simulink model "SoftwareArchitecture"  (R2024a)
settings: Solver=FixedStepDiscrete  StartTime=0.0  StopTime=10.0  RelTol=1e-3
settings Model: Creator=njsne  LastModifiedBy=njsne

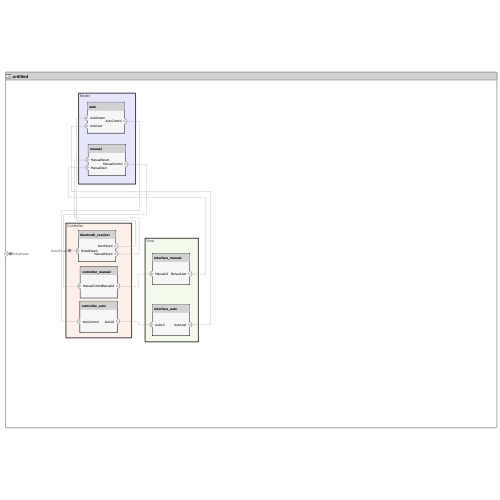
[thumbnail: Simulink's stored preview of the top-level diagram]
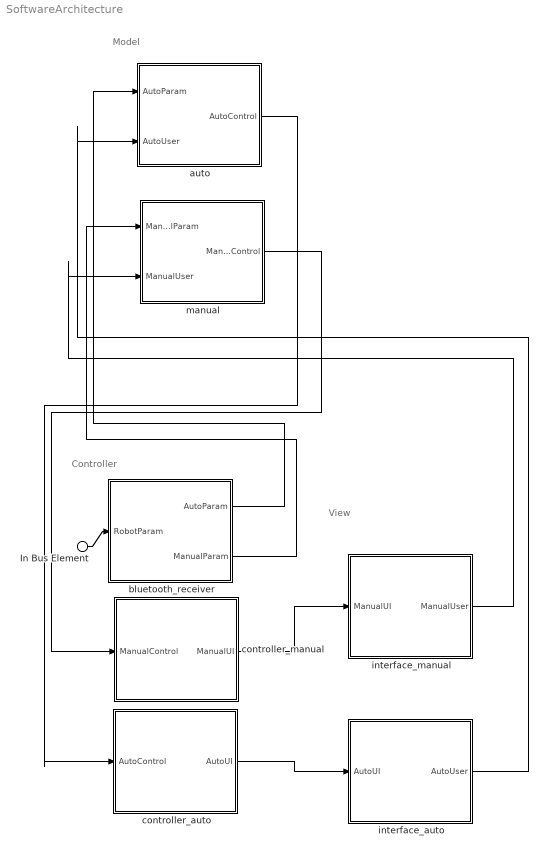
== system SoftwareArchitecture ==
  note: Model
  note: Controller
  note: View
  In Bus Element : Inport  PortName=RobotParam
  auto : Subsystem
      settings: PortSchema="{\"entries\":[{\"content\":{\"headerSize\":26,\"margin\":15,\"minimumSpacing\":25,\"sides\":[{\"content\":{\"connectorIds\":[\"In1\",\"In2\"]},\"type\":\"ConnectorPlacement.EquallySpacedRectSide\",\"uuid\":\"f355d6d0-cf58-497d-af4c-3e4dcc6a73b6\"},{\"content\":{\"connectorIds\":[\"Out1\"],\"side\":\"RIGHT\"},\"type\":\"ConnectorPlacement.EquallySpacedRectSide\",\"uuid\":\"26958e8c-f185-4cf9-b08a-6b963fcd1ab7\"},{\"content\":{\"side\":\"TOP\"},\"type\":\"ConnectorPlacement.EquallySpacedRectSide\",\"uuid\":\"bb7e5bb3-6807-4390-828c-0753e6f4db2d\"}]},\"type\":\"ConnectorPlacement.EquallySpacedConnector\",\"uuid\":\"9cb3c599-3bd4-42ed-97e1-2535c9f88a3a\"}],\"packageUris\":[\"http://schema.mathworks.com/mf0/Connector/R2020b\"],\"version\":\"1.0\"}"
  bluetooth_receiver : Subsystem
      settings: PortSchema="{\"entries\":[{\"content\":{\"headerSize\":26,\"margin\":15,\"minimumSpacing\":25,\"sides\":[{\"content\":{\"connectorIds\":[\"In1\"]},\"type\":\"ConnectorPlacement.EquallySpacedRectSide\",\"uuid\":\"f355d6d0-cf58-497d-af4c-3e4dcc6a73b6\"},{\"content\":{\"connectorIds\":[\"Out1\",\"Out2\"],\"side\":\"RIGHT\"},\"type\":\"ConnectorPlacement.EquallySpacedRectSide\",\"uuid\":\"26958e8c-f185-4cf9-b08a-6b963fcd1ab7\"},{\"content\":{\"side\":\"TOP\"},\"type\":\"ConnectorPlacement.EquallySpacedRectSide\",\"uuid\":\"bb7e5bb3-6807-4390-828c-0753e6f4db2d\"}]},\"type\":\"ConnectorPlacement.EquallySpacedConnector\",\"uuid\":\"9cb3c599-3bd4-42ed-97e1-2535c9f88a3a\"}],\"packageUris\":[\"http://schema.mathworks.com/mf0/Connector/R2020b\"],\"version\":\"1.0\"}"
  controller_auto : Subsystem
      settings: PortSchema="{\"entries\":[{\"content\":{\"headerSize\":26,\"margin\":15,\"minimumSpacing\":25,\"sides\":[{\"content\":{\"connectorIds\":[\"In1\"]},\"type\":\"ConnectorPlacement.EquallySpacedRectSide\",\"uuid\":\"f355d6d0-cf58-497d-af4c-3e4dcc6a73b6\"},{\"content\":{\"connectorIds\":[\"Out1\"],\"side\":\"RIGHT\"},\"type\":\"ConnectorPlacement.EquallySpacedRectSide\",\"uuid\":\"26958e8c-f185-4cf9-b08a-6b963fcd1ab7\"},{\"content\":{\"side\":\"TOP\"},\"type\":\"ConnectorPlacement.EquallySpacedRectSide\",\"uuid\":\"bb7e5bb3-6807-4390-828c-0753e6f4db2d\"}]},\"type\":\"ConnectorPlacement.EquallySpacedConnector\",\"uuid\":\"9cb3c599-3bd4-42ed-97e1-2535c9f88a3a\"}],\"packageUris\":[\"http://schema.mathworks.com/mf0/Connector/R2020b\"],\"version\":\"1.0\"}"
  controller_manual : Subsystem
      settings: PortSchema="{\"entries\":[{\"content\":{\"headerSize\":26,\"margin\":15,\"minimumSpacing\":25,\"sides\":[{\"content\":{\"connectorIds\":[\"In1\"]},\"type\":\"ConnectorPlacement.EquallySpacedRectSide\",\"uuid\":\"f355d6d0-cf58-497d-af4c-3e4dcc6a73b6\"},{\"content\":{\"connectorIds\":[\"Out1\"],\"side\":\"RIGHT\"},\"type\":\"ConnectorPlacement.EquallySpacedRectSide\",\"uuid\":\"26958e8c-f185-4cf9-b08a-6b963fcd1ab7\"},{\"content\":{\"side\":\"TOP\"},\"type\":\"ConnectorPlacement.EquallySpacedRectSide\",\"uuid\":\"bb7e5bb3-6807-4390-828c-0753e6f4db2d\"}]},\"type\":\"ConnectorPlacement.EquallySpacedConnector\",\"uuid\":\"9cb3c599-3bd4-42ed-97e1-2535c9f88a3a\"}],\"packageUris\":[\"http://schema.mathworks.com/mf0/Connector/R2020b\"],\"version\":\"1.0\"}"
  interface_auto : Subsystem
      settings: PortSchema="{\"entries\":[{\"content\":{\"headerSize\":26,\"margin\":15,\"minimumSpacing\":25,\"sides\":[{\"content\":{\"connectorIds\":[\"In1\"]},\"type\":\"ConnectorPlacement.EquallySpacedRectSide\",\"uuid\":\"f355d6d0-cf58-497d-af4c-3e4dcc6a73b6\"},{\"content\":{\"connectorIds\":[\"Out1\"],\"side\":\"RIGHT\"},\"type\":\"ConnectorPlacement.EquallySpacedRectSide\",\"uuid\":\"26958e8c-f185-4cf9-b08a-6b963fcd1ab7\"},{\"content\":{\"side\":\"TOP\"},\"type\":\"ConnectorPlacement.EquallySpacedRectSide\",\"uuid\":\"bb7e5bb3-6807-4390-828c-0753e6f4db2d\"}]},\"type\":\"ConnectorPlacement.EquallySpacedConnector\",\"uuid\":\"9cb3c599-3bd4-42ed-97e1-2535c9f88a3a\"}],\"packageUris\":[\"http://schema.mathworks.com/mf0/Connector/R2020b\"],\"version\":\"1.0\"}"
  interface_manual : Subsystem
      settings: PortSchema="{\"entries\":[{\"content\":{\"headerSize\":26,\"margin\":15,\"minimumSpacing\":25,\"sides\":[{\"content\":{\"connectorIds\":[\"In1\"]},\"type\":\"ConnectorPlacement.EquallySpacedRectSide\",\"uuid\":\"f355d6d0-cf58-497d-af4c-3e4dcc6a73b6\"},{\"content\":{\"connectorIds\":[\"Out1\"],\"side\":\"RIGHT\"},\"type\":\"ConnectorPlacement.EquallySpacedRectSide\",\"uuid\":\"26958e8c-f185-4cf9-b08a-6b963fcd1ab7\"},{\"content\":{\"side\":\"TOP\"},\"type\":\"ConnectorPlacement.EquallySpacedRectSide\",\"uuid\":\"bb7e5bb3-6807-4390-828c-0753e6f4db2d\"}]},\"type\":\"ConnectorPlacement.EquallySpacedConnector\",\"uuid\":\"9cb3c599-3bd4-42ed-97e1-2535c9f88a3a\"}],\"packageUris\":[\"http://schema.mathworks.com/mf0/Connector/R2020b\"],\"version\":\"1.0\"}"
  manual : Subsystem
      settings: PortSchema="{\"entries\":[{\"content\":{\"headerSize\":26,\"margin\":15,\"minimumSpacing\":25,\"sides\":[{\"content\":{\"connectorIds\":[\"In1\",\"In2\"]},\"type\":\"ConnectorPlacement.EquallySpacedRectSide\",\"uuid\":\"f355d6d0-cf58-497d-af4c-3e4dcc6a73b6\"},{\"content\":{\"connectorIds\":[\"Out1\"],\"side\":\"RIGHT\"},\"type\":\"ConnectorPlacement.EquallySpacedRectSide\",\"uuid\":\"26958e8c-f185-4cf9-b08a-6b963fcd1ab7\"},{\"content\":{\"side\":\"TOP\"},\"type\":\"ConnectorPlacement.EquallySpacedRectSide\",\"uuid\":\"bb7e5bb3-6807-4390-828c-0753e6f4db2d\"}]},\"type\":\"ConnectorPlacement.EquallySpacedConnector\",\"uuid\":\"9cb3c599-3bd4-42ed-97e1-2535c9f88a3a\"}],\"packageUris\":[\"http://schema.mathworks.com/mf0/Connector/R2020b\"],\"version\":\"1.0\"}"
  wires:
  bluetooth_receiver/1(AutoParam) -> auto/1(AutoParam)
  bluetooth_receiver/2(ManualParam) -> manual/1(ManualParam)
  auto/1(AutoControl) -> controller_auto/1(AutoControl)
  controller_auto/1(AutoUI) -> interface_auto/1(AutoUI)
  interface_manual/1(ManualUser) -> manual/2(ManualUser)
  manual/1(ManualControl) -> controller_manual/1(ManualControl)
  controller_manual/1(ManualUI) -> interface_manual/1(ManualUI)
  interface_auto/1(AutoUser) -> auto/2(AutoUser)
  In Bus Element/1 -> bluetooth_receiver/1(RobotParam)

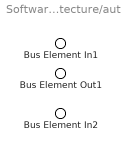
== system SoftwareArchitecture/auto ==
  Bus Element In1 : Inport  PortName=AutoParam
  Bus Element In2 : Inport  Port=2  PortName=AutoUser
  Bus Element Out1 : Outport  PortName=AutoControl

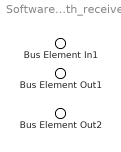
== system SoftwareArchitecture/bluetooth_receiver ==
  Bus Element In1 : Inport  PortName=RobotParam
  Bus Element Out1 : Outport  PortName=AutoParam
  Bus Element Out2 : Outport  Port=2  PortName=ManualParam

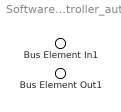
== system SoftwareArchitecture/controller_auto ==
  Bus Element In1 : Inport  PortName=AutoControl
  Bus Element Out1 : Outport  PortName=AutoUI

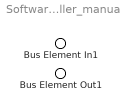
== system SoftwareArchitecture/controller_manual ==
  Bus Element In1 : Inport  PortName=ManualControl
  Bus Element Out1 : Outport  PortName=ManualUI

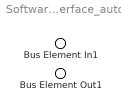
== system SoftwareArchitecture/interface_auto ==
  Bus Element In1 : Inport  PortName=AutoUI
  Bus Element Out1 : Outport  PortName=AutoUser

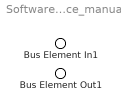
== system SoftwareArchitecture/interface_manual ==
  Bus Element In1 : Inport  PortName=ManualUI
  Bus Element Out1 : Outport  PortName=ManualUser

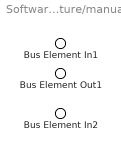
== system SoftwareArchitecture/manual ==
  Bus Element In1 : Inport  PortName=ManualParam
  Bus Element In2 : Inport  Port=2  PortName=ManualUser
  Bus Element Out1 : Outport  PortName=ManualControl
